simulink model "tanques_nl"  (R2018a)
settings: Solver=VariableStepAuto  StartTime=0.0  StopTime=t(end)+10  RelTol=1e-3
InitFcn:
  | tanques_lineal_non_lineal
values from neighbouring files (symbols this model uses):
  A = 10    [tanques_lineal_non_lineal.m]
  Aj = double(Aj)    [tanques_lineal_non_lineal.m]
  Bj = double(Bj)    [tanques_lineal_non_lineal.m]
  h1e = 2*h2e    [tanques_lineal_non_lineal.m]
  h2e = (Q/k)^2    [tanques_lineal_non_lineal.m]
  k = As*sqrt(2*g)    [tanques_lineal_non_lineal.m]
  q = 0.01    [tanques_lineal_non_lineal.m]
  Q = 2    [tanques_lineal_non_lineal.m]
  X0 = 1.1*Xe    [tanques_lineal_non_lineal.m]
  Xini = X0-Xe    [tanques_lineal_non_lineal.m]
settings Model: Creator=carma  LastModifiedBy=carma

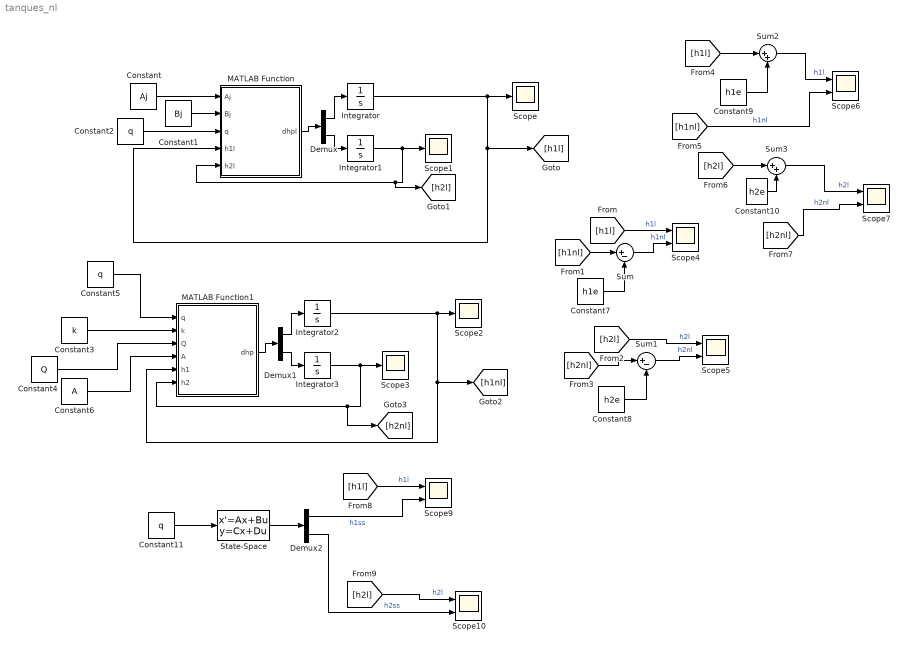
== system tanques_nl ==
  Constant : Constant  Value=Aj
  Constant1 : Constant  Value=Bj
  Constant10 : Constant  Value=h2e
  Constant11 : Constant  Value=q
  Constant2 : Constant  Value=q
  Constant3 : Constant  Value=k
  Constant4 : Constant  Value=Q
  Constant5 : Constant  Value=q
  Constant6 : Constant  Value=A
  Constant7 : Constant  Value=h1e
  Constant8 : Constant  Value=h2e
  Constant9 : Constant  Value=h1e
  Demux : Demux  Outputs=2
  Demux1 : Demux  Outputs=2
  Demux2 : Demux  Outputs=2
  Integrator : Integrator  InitialCondition=Xini(1,1)
  Integrator1 : Integrator  InitialCondition=Xini(1,2)
  Integrator2 : Integrator  InitialCondition=X0(1,1)
  Integrator3 : Integrator  InitialCondition=X0(1,2)
  MATLAB Function : MATLAB Function  TreatAsAtomicUnit=on
  MATLAB Function1 : MATLAB Function  TreatAsAtomicUnit=on
  Scope{,1..3} (4 alike) : Scope
  Scope{4..7,9..10} (6 alike) : Scope  NumInputPorts=2
  State-Space : StateSpace  A=Aj  B=Bj  C=eye(2)  D=zeros(2,1)  InitialCondition=Xini
  Sum : Sum  Inputs=|+-
  Sum1 : Sum  Inputs=|+-
  Sum2 : Sum  Inputs=|++
  Sum3 : Sum  Inputs=|++
  wires:
  Integrator/1 -> [h1l], MATLAB Function/4(h1l), Scope/1
  MATLAB Function/1(dhpl) -> Demux/1
  Constant/1 -> MATLAB Function/1(Aj)
  Constant1/1 -> MATLAB Function/2(Bj)
  Constant2/1 -> MATLAB Function/3(q)
  Demux/1 -> Integrator/1
  Demux/2 -> Integrator1/1
  Integrator3/1 -> [h2nl], MATLAB Function1/6(h2), Scope3/1
  Constant3/1 -> MATLAB Function1/2(k)
  Constant4/1 -> MATLAB Function1/3(Q)
  Integrator2/1 -> [h1nl], MATLAB Function1/5(h1), Scope2/1
  Demux1/2 -> Integrator3/1
  MATLAB Function1/1(dhp) -> Demux1/1
  Constant5/1 -> MATLAB Function1/1(q)
  Demux1/1 -> Integrator2/1
  Constant6/1 -> MATLAB Function1/4(A)
  Integrator1/1 -> [h2l], MATLAB Function/5(h2l), Scope1/1
  [h1l] -> Scope4/1  "h1l"
  [h1nl] -> Sum/1
  Sum/1 -> Scope4/2  "h1nl"
  Constant7/1 -> Sum/2
  Constant8/1 -> Sum1/2
  Sum1/1 -> Scope5/2  "h2nl"
  [h2l] -> Scope5/1  "h2l"
  [h2nl] -> Sum1/1
  [h1nl] -> Scope6/2  "h1nl"
  [h2nl] -> Scope7/2  "h2nl"
  Constant9/1 -> Sum2/2
  [h1l] -> Sum2/1
  Sum2/1 -> Scope6/1  "h1l"
  Constant10/1 -> Sum3/2
  [h2l] -> Sum3/1
  Sum3/1 -> Scope7/1  "h2l"
  Constant11/1 -> State-Space/1
  [h1l] -> Scope9/1  "h1l"
  [h2l] -> Scope10/1  "h2l"
  State-Space/1 -> Demux2/1
  Demux2/1 -> Scope9/2  "h1ss"
  Demux2/2 -> Scope10/2  "h2ss"

== matlab function tanques_nl/MATLAB Function1 ==
  data: q input; k input; Q input; dhp output; A input; h1 input; h2 input
function dhp  = fcn(q,k,Q,A,h1,h2)

q1=Q+q; %Entrada del sistema



q12=k*sqrt(abs(h1-h2));
q2=k*sqrt(h2);
h1p=(q1-q12)/A;
h2p=(q12-q2)/A;

dhp=[h1p;h2p];

== matlab function tanques_nl/MATLAB Function ==
  data: Aj input; Bj input; q input; dhpl output; h1l input; h2l input
function dhpl   = fcn(Aj,Bj,q,h1l,h2l)

h=[h1l ; h2l];
dhpl=Aj*h+Bj*q;
